simulink model "ts_adapt_const"  (R2020b)
settings: Solver=ode1  StartTime=0.0  StopTime=70  FixedStep=0.001  RelTol=1e-3
undefined symbols (not defined in the file or in its folder): Serial_Port, Standard_Devices
libraries: sldrtlib x2
settings Model: ExtModeTrigDuration=120000  Creator=Mesih  LastModifiedBy=Mesih
settings RTWCC: Description=Simulink Desktop Real-Time  SystemTargetFile=sldrt.tlc  TemplateMakefile=sldrt.tmf  RTWCompilerOptimization=on
settings CodeAppCC: MaxIdLength=95
settings SimulinkDesktopRealTimeCC: TargetPreCompLibLocation=C:\Program Files\MATLAB\R2020b\toolbox\sldrt\lib\win64

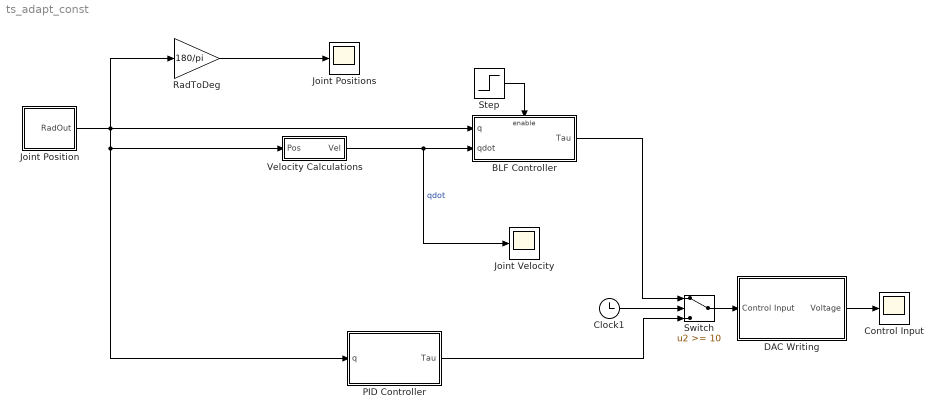
== system ts_adapt_const ==
  BLF Controller : Subsystem  TreatAsAtomicUnit=on
  Clock1 : Clock
  Control Input : Scope
  DAC Writing : Subsystem
  Joint Position : Subsystem
  Joint Positions : Scope
  Joint Velocity : Scope
  PID Controller : Subsystem
  RadToDeg : Gain  Gain=180/pi
  Step : Step  Time=10
  Switch : Switch  Threshold=10
  Velocity Calculations : Subsystem
  wires:
  DAC Writing/1(Voltage) -> Control Input/1
  Joint Position/1(RadOut) -> PID Controller/1(q), Velocity Calculations/1(Pos), RadToDeg/1, BLF Controller/1(q)
  Switch/1 -> DAC Writing/1(Control Input)
  Clock1/1 -> Switch/2
  RadToDeg/1 -> Joint Positions/1
  Velocity Calculations/1(Vel) -> BLF Controller/2(qdot), Joint Velocity/1  "qdot"
  BLF Controller/1(Tau) -> Switch/1
  Step/1 -> BLF Controller/Enable
  PID Controller/1(Tau) -> Switch/3

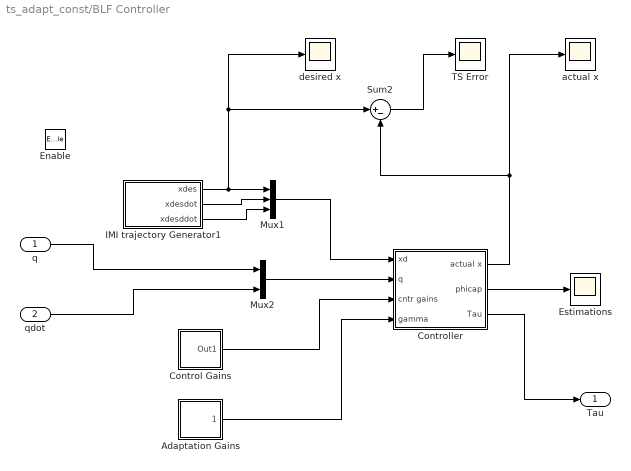
== system ts_adapt_const/BLF Controller ==
  q : Inport
  qdot : Inport  Port=2
  Enable : EnablePort
  Adaptation Gains : Subsystem
  Control Gains : Subsystem
  Controller : Subsystem
  Estimations : Scope
  IMI trajectory Generator1 : Subsystem  mask{ampl=[0.05 0.04], freq=[1.0 1.0]}
      mask prompts: ampl "Amplitute"; freq "Frequency"
  Mux1 : Mux  Inputs=3
  Mux2 : Mux  Inputs=2
  Sum2 : Sum  Inputs=|+-
  TS Error : Scope
  actual x : Scope
  desired x : Scope
  Tau : Outport
  wires:
  Controller/3(Tau) -> Tau/1
  Control Gains/1(Out1) -> Controller/3(cntr gains)
  Adaptation Gains/1(gamma) -> Controller/4(gamma)
  Mux2/1 -> Controller/2(q)
  Controller/1(actual x) -> actual x/1, Sum2/2
  Controller/2(phicap) -> Estimations/1
  Sum2/1 -> TS Error/1
  IMI trajectory Generator1/1(xdes) -> Mux1/1, Sum2/1, desired x/1
  Mux1/1 -> Controller/1(xd)
  q/1 -> Mux2/1
  IMI trajectory Generator1/2(xdesdot) -> Mux1/2
  qdot/1 -> Mux2/2
  IMI trajectory Generator1/3(xdesddot) -> Mux1/3

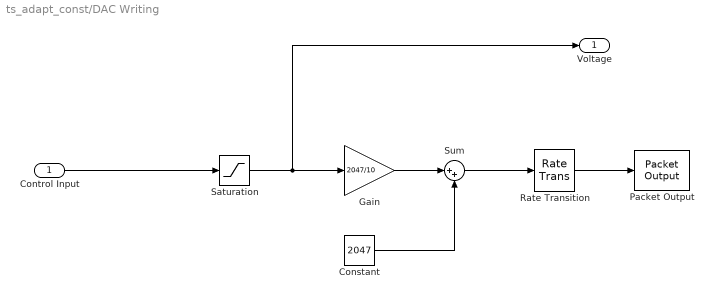
== system ts_adapt_const/DAC Writing ==
  Control Input : Inport
  Constant : Constant  Value=2047
  Gain : Gain  Gain=2047/10
  Packet Output : sldrtlib/Packet Output  SampleTime=-1  MaxMissedTicks=1  ShowMissedTicks=off  YieldWhenWaiting=on  DrvName=Standard_Devices/Serial_Port  DrvAddress=6  DrvOptions=[256000 8 0 0 0 0 0 0]  PacketSize=6  DataTypes='3*uint16'  ShowReady=off  ShowError=off  PacketID=1  ByteOrder=1  InitialValue=[]  FinalValue=[]
      settings: AttributesFormatString=Serial Port [6]
  Rate Transition : RateTransition  Deterministic=off  OutPortSampleTimeOpt=Inherit
  Saturation : Saturate  UpperLimit=10  LowerLimit=-10
  Sum : Sum  Inputs=|++
  Voltage : Outport
  wires:
  Rate Transition/1 -> Packet Output/1
  Saturation/1 -> Voltage/1, Gain/1
  Gain/1 -> Sum/1
  Sum/1 -> Rate Transition/1
  Constant/1 -> Sum/2
  Control Input/1 -> Saturation/1

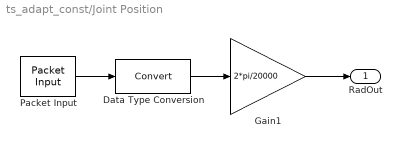
== system ts_adapt_const/Joint Position ==
  Data Type Conversion : DataTypeConversion
  Gain1 : Gain  Gain=2*pi/20000
  Packet Input : sldrtlib/Packet Input  SampleTime=-1  MaxMissedTicks=1  ShowMissedTicks=off  YieldWhenWaiting=on  DrvName=Standard_Devices/Serial_Port  DrvAddress=6  DrvOptions=[256000 8 0 0 0 0 0 0]  PacketSize=6  DataTypes='3*int16'  ShowReady=off  ShowError=off  PacketID=1  ByteOrder=1  ShowTimestamp=off
      settings: AttributesFormatString=Serial Port [6]
  RadOut : Outport
  wires:
  Gain1/1 -> RadOut/1
  Data Type Conversion/1 -> Gain1/1
  Packet Input/1 -> Data Type Conversion/1

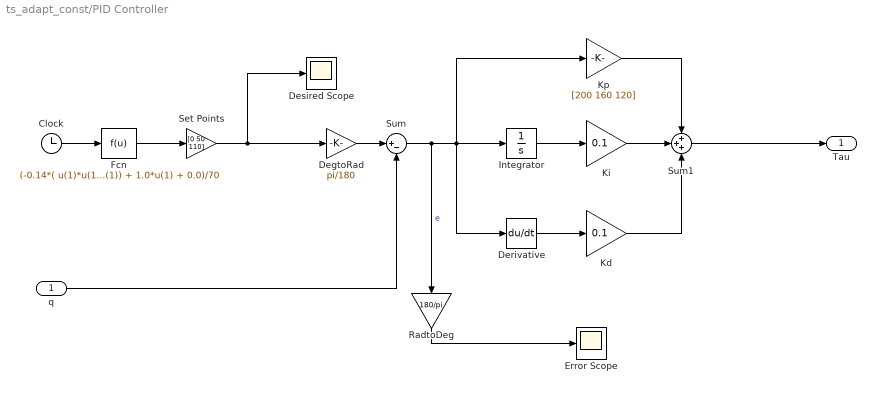
== system ts_adapt_const/PID Controller ==
  q : Inport
  Clock : Clock
  DegtoRad : Gain  Gain=pi/180
  Derivative : Derivative
  Desired Scope : Scope
  Error Scope : Scope
  Fcn : Fcn  Expr=(-0.14*( u(1)*u(1)*u(1)) + 2.0*( u(1)*u(1)) + 1.0*u(1) + 0.0)/70
  Integrator : Integrator
  Kd : Gain  Gain=0.1
  Ki : Gain  Gain=0.1
  Kp : Gain  Gain=[200 160 120]
  RadtoDeg : Gain  Gain=180/pi
  Set Points : Gain  Gain=[0 50 110]
  Sum : Sum  Inputs=|+-
  Sum1 : Sum  Inputs=+++
  Tau : Outport
  wires:
  Set Points/1 -> Desired Scope/1, DegtoRad/1
  Kp/1 -> Sum1/1
  Integrator/1 -> Ki/1
  Clock/1 -> Fcn/1
  Derivative/1 -> Kd/1
  Fcn/1 -> Set Points/1
  Sum/1 -> Integrator/1, Kp/1, Derivative/1, RadtoDeg/1  "e"
  Kd/1 -> Sum1/3
  DegtoRad/1 -> Sum/1
  RadtoDeg/1 -> Error Scope/1
  Ki/1 -> Sum1/2
  Sum1/1 -> Tau/1
  q/1 -> Sum/2

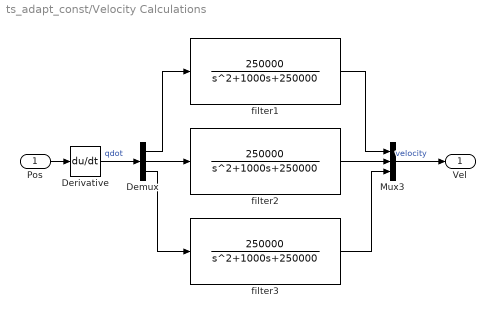
== system ts_adapt_const/Velocity Calculations ==
  Pos : Inport
  Demux : Demux  Outputs=3
  Derivative : Derivative
  Mux3 : Mux  Inputs=3
  filter1 : TransferFcn  Numerator=[250000]  Denominator=[1 1000 250000]
  filter2 : TransferFcn  Numerator=[250000]  Denominator=[1 1000 250000]
  filter3 : TransferFcn  Numerator=[250000]  Denominator=[1 1000 250000]
  Vel : Outport
  wires:
  Demux/2 -> filter2/1
  filter1/1 -> Mux3/1
  Derivative/1 -> Demux/1  "qdot"
  Pos/1 -> Derivative/1
  Mux3/1 -> Vel/1  "velocity"
  Demux/1 -> filter1/1
  filter2/1 -> Mux3/2
  Demux/3 -> filter3/1
  filter3/1 -> Mux3/3

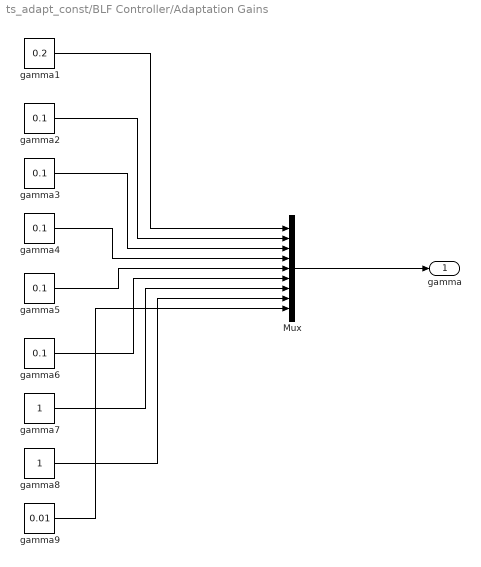
== system ts_adapt_const/BLF Controller/Adaptation Gains ==
  Mux : Mux  Inputs=9
  gamma1 : Constant  Value=0.2
  gamma{2..6} (5 alike) : Constant  Value=0.1
  gamma7 : Constant
  gamma8 : Constant
  gamma9 : Constant  Value=0.01
  gamma : Outport
  wires:
  gamma1/1 -> Mux/1
  Mux/1 -> gamma/1
  gamma4/1 -> Mux/4
  gamma3/1 -> Mux/3
  gamma2/1 -> Mux/2
  gamma5/1 -> Mux/5
  gamma6/1 -> Mux/6
  gamma7/1 -> Mux/7
  gamma8/1 -> Mux/8
  gamma9/1 -> Mux/9

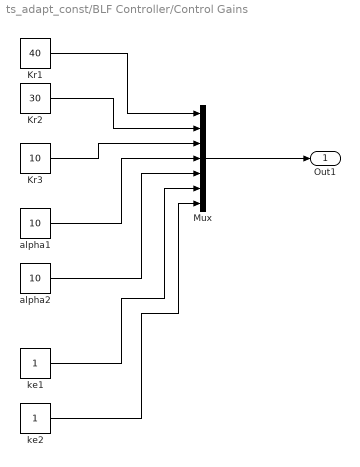
== system ts_adapt_const/BLF Controller/Control Gains ==
  Kr1 : Constant  Value=40
  Kr2 : Constant  Value=30
  Kr3 : Constant  Value=10
  Mux : Mux  Inputs=7
  alpha1 : Constant  Value=10
  alpha2 : Constant  Value=10
  ke1 : Constant
  ke2 : Constant
  Out1 : Outport
  wires:
  Kr1/1 -> Mux/1
  Mux/1 -> Out1/1
  Kr2/1 -> Mux/2
  Kr3/1 -> Mux/3
  alpha1/1 -> Mux/4
  alpha2/1 -> Mux/5
  ke2/1 -> Mux/7
  ke1/1 -> Mux/6

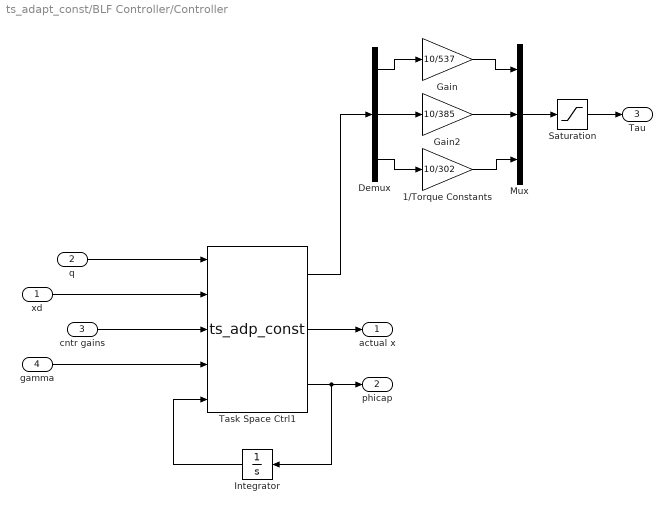
== system ts_adapt_const/BLF Controller/Controller ==
  xd : Inport
  q : Inport  Port=2
  cntr gains : Inport  Port=3
  gamma : Inport  Port=4
  1/Torque Constants : Gain  Gain=10/302
  Demux : Demux  Outputs=3
  Gain : Gain  Gain=10/537
  Gain2 : Gain  Gain=10/385
  Integrator : Integrator
  Mux : Mux  Inputs=3
  Saturation : Saturate  UpperLimit=10  LowerLimit=-10
  Task Space Ctrl1 : S-Function  FunctionName=ts_adp_const  SFunctionDeploymentMode=off  EnableBusSupport=off
  actual x : Outport
  phicap : Outport  Port=2
  Tau : Outport  Port=3
  wires:
  Integrator/1 -> Task Space Ctrl1/5
  cntr gains/1 -> Task Space Ctrl1/3
  Task Space Ctrl1/3 -> phicap/1, Integrator/1
  q/1 -> Task Space Ctrl1/1
  Task Space Ctrl1/2 -> actual x/1
  xd/1 -> Task Space Ctrl1/2
  gamma/1 -> Task Space Ctrl1/4
  Task Space Ctrl1/1 -> Demux/1
  1/Torque Constants/1 -> Mux/3
  Demux/2 -> Gain2/1
  Demux/1 -> Gain/1
  Demux/3 -> 1/Torque Constants/1
  Gain/1 -> Mux/1
  Gain2/1 -> Mux/2
  Mux/1 -> Saturation/1
  Saturation/1 -> Tau/1

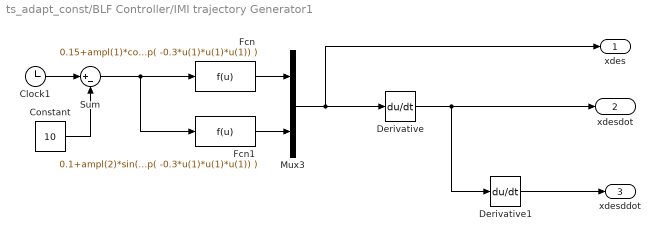
== system ts_adapt_const/BLF Controller/IMI trajectory Generator1 ==
  Clock1 : Clock
  Constant : Constant  Value=10
  Derivative : Derivative
  Derivative1 : Derivative
  Fcn : Fcn  Expr=0.15+ampl(1)*cos(freq(1)*u(1))*( 1-exp( -0.3*u(1)*u(1)*u(1)) )
  Fcn1 : Fcn  Expr=0.1+ampl(2)*sin(freq(2)*u(1))*( 1-exp( -0.3*u(1)*u(1)*u(1)) )
  Mux3 : Mux  Inputs=2
  Sum : Sum  Inputs=|+-
  xdes : Outport  VectorParamsAs1DForOutWhenUnconnected=off
  xdesdot : Outport  Port=2  VectorParamsAs1DForOutWhenUnconnected=off
  xdesddot : Outport  Port=3
  wires:
  Fcn/1 -> Mux3/1
  Fcn1/1 -> Mux3/2
  Mux3/1 -> Derivative/1, xdes/1
  Derivative/1 -> Derivative1/1, xdesdot/1
  Derivative1/1 -> xdesddot/1
  Clock1/1 -> Sum/1
  Sum/1 -> Fcn1/1, Fcn/1
  Constant/1 -> Sum/2
